simulink model "inner_pd_continuous_test"  (R2016b)
settings: Solver=VariableStepAuto  StartTime=0.0  StopTime=30  RelTol=1e-3  EnableMultiTasking=on
values from neighbouring files (symbols this model uses):
  max_ang_ref = pi/8    (= 0.392699081699)    [init.m]
  omega_max_lim = 2500    [init.m]
  omega_min_lim = 0    [init.m]
  T_max_lim = Tp - (Tp - Tm) * sat_lim    [init.m]
  tau_max_lim = 1e-5    (= 1e-05)    [init.m]
  tau_min_lim = -1e-5    (= -1e-05)    [init.m]
undefined symbols (not defined in the file or in its folder): inner_h, k
libraries: simulink x3, vrlib x2
settings Model: Creator=Daniel  LastModifiedBy=abhijit
settings DataIOCC: LimitDataPoints=on
settings OptimizationCC: LifeSpan=inf
settings DebuggingCC: AllowSymbolicDim=off  SFUnexpectedBacktrackingDiag=warning  SFNoUnconditionalDefaultTransitionDiag=warning  SFExecutionAtInitializationDiag=none
settings ModelReferenceCC: PropagateSignalLabelsOutOfModel=off
settings GRTTargetCC: TargetLangStandard=C89/C90 (ANSI)
settings ConfigComp: CovMetricSettings=dw  CovHtmlReporting=on  CovSaveCumulativeToWorkspaceVar=on  CovSaveSingleToWorkspaceVar=on  CovExternalEMLEnable=off

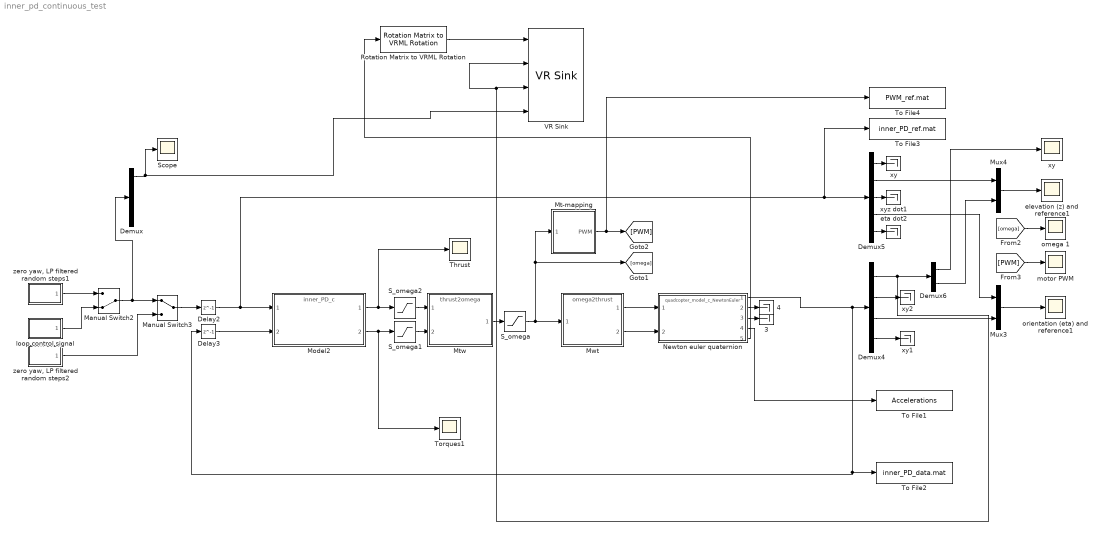
== system inner_pd_continuous_test ==
  "   3" : Terminator
  "   4" : Terminator
  "   eta dot2" : Terminator
  "   xy" : Terminator
  "   xy1" : Terminator
  "   xy2" : Terminator
  "  xyz dot1" : Terminator
  Delay2 : Delay  DelayLength=1  InitialCondition=0  SampleTime=inner_h
  Delay3 : Delay  DelayLength=1  InitialCondition=0  SampleTime=inner_h
  Demux : Demux
  Demux4 : Demux  Outputs=[3,3,3,3]
  Demux5 : Demux  Outputs=[2,1,3,3,3]
  Demux6 : Demux  Outputs=[2,1]
  Manual Switch2 : ManualSwitch  CurrentSetting=0
  Manual Switch3 : ManualSwitch
  Model2 : ModelReference  ModelNameDialog=inner_PD_c.mdl  SimulationMode=Normal  ModelReferenceVersion=1.87
  Mt-mapping : Subsystem
  Mtw : ModelReference  ModelNameDialog=thrust2omega.mdl  SimulationMode=Normal  ModelReferenceVersion=1.3
  Mux3 : Mux  Inputs=2
  Mux4 : Mux  Inputs=2
  Mwt : ModelReference  ModelNameDialog=omega2thrust.mdl  SimulationMode=Normal  ModelReferenceVersion=1.3
  Newton euler quaternion : ModelReference  ModelNameDialog=quadcopter_model_c_NewtonEuler.mdl  SimulationMode=Normal  ModelReferenceVersion=1.327
  Rotation Matrix to VRML Rotation : vrlib/Utilities/Rotation Matrix to VRML Rotation  maxzero=1e-12
  S_omega : Saturate  UpperLimit=omega_max_lim  LowerLimit=omega_min_lim
  S_omega1 : Saturate  UpperLimit=tau_max_lim  LowerLimit=tau_min_lim
  S_omega2 : Saturate  UpperLimit=T_max_lim  LowerLimit=tau_min_lim
  Scope : Scope
  Thrust : Scope
  To File1 : ToFile  Filename=Accelerations  MatrixName=Accel  SaveFormat=Timeseries  SampleTime=inner_h
  To File2 : ToFile  Filename=inner_PD_data.mat  MatrixName=PD_data  SaveFormat=Timeseries  SampleTime=inner_h
  To File3 : ToFile  Filename=inner_PD_ref.mat  MatrixName=PD_ref  SaveFormat=Timeseries  SampleTime=inner_h
  To File4 : ToFile  Filename=PWM_ref.mat  MatrixName=PWM  SaveFormat=Timeseries  SampleTime=inner_h
  Torques1 : Scope
  VR Sink : vrlib/VR Sink  InstantiateOnLoad=on  SampleTime=0.05  ViewEnable=on  RemoteChange=off  RemoteView=off  FieldsWritten=copter.rotation.4.1.1.double#copter.translation.3.1.1.double#vp.translation.3.1.1.double#target.translation.3.1.1.double  WorldFileName=copter_world.wrl  WorldDescription=quadcopter_world  AutoView=on  VideoDimensions=[]  AllowVariableSize=off  FigureProperties="{'Position', 'Name', 'Viewpoint', 'CameraBound', 'CameraDirection', 'CameraPosition', 'CameraUpVector', 'ZoomFactor', 'Antialiasing', 'Headlight', 'Lighting', 'NavPanel', 'Sound', 'StatusBar', 'Stereo3D', 'Stereo3DCameraOffset', 'Stereo3DHIT', 'ToolBar', 'Textures', 'Transparency', 'Triad', 'Wireframe', 'NavZones', 'NavMode', 'NavSpeed', 'CaptureFileFormat', 'CaptureFileName', 'Record2DCompressMethod', 'Record2DCompressQuality', 'Record2D', 'Record2DFileName', 'Record2DFPS'; [7.6000000000000000e+01   1.1600000000000000e+02   5.7600000000000000e+02   3.5000000000000000e+02], 'quadcopter_world', 'viewpoint', 'on', [0.0000000000000000e+00   0.0000000000000000e+00  -1.0000000000000000e+00], [0.0000000000000000e+00   0.0000000000000000e+00   0.0000000000000000e+00], [0.0000000000000000e+00   1.0000000000000000e+00   0.0000000000000000e+00], [1.0000000000000000e+00], 'on', 'on', 'on', 'halfbar', 'on', 'on', 'off', [1.0000000149011612e-01], [0.0000000000000000e+00], 'on', 'on', 'on', 'none', 'off', 'off', 'fly', 'normal', 'tif', '%f_anim_%n.tif', 'auto', [7.5000000000000000e+01], 'off', '%f_anim_%n.avi', 'auto'}"
  elevation (z) and reference1 : Scope
  loop control signal : Subsystem
  motor PWM : Scope
  omega 1 : Scope
  orientation (eta) and reference1 : Scope
  xy : Scope
  "zero yaw, LP filtered random steps1" : Subsystem
  "zero yaw, LP filtered random steps2" : Subsystem
  wires:
  loop control signal/1(reference) -> Manual Switch2/2
  "zero yaw, LP filtered random steps1"/1(reference) -> Manual Switch2/1
  Demux5/2 -> Mux4/1
  Mux4/1 -> elevation (z) and reference1/1
  Newton euler quaternion/1 -> Delay3/1, To File2/1, Demux4/1
  Mux3/1 -> orientation (eta) and reference1/1
  Demux5/3 -> "  xyz dot1"/1
  Demux5/5 -> "   eta dot2"/1
  Demux5/1 -> "   xy"/1
  Demux4/3 -> Mux3/2
  Demux4/1 -> VR Sink/2, VR Sink/3, Demux6/1
  [omega] -> omega 1/1
  Demux5/4 -> Mux3/1
  Delay2/1 -> Model2/1, To File3/1, Demux5/1
  Demux4/4 -> "   xy1"/1
  Demux4/2 -> "   xy2"/1
  Demux6/2 -> Mux4/2
  Demux6/1 -> xy/1
  Mt-mapping/1(PWM) -> [PWM], To File4/1
  [PWM] -> motor PWM/1
  Manual Switch2/1 -> Demux/1, Manual Switch3/1
  Manual Switch3/1 -> Delay2/1
  "zero yaw, LP filtered random steps2"/1(reference) -> Manual Switch3/2
  Newton euler quaternion/3 -> "   3"/1
  Newton euler quaternion/2 -> "   4"/1
  Mtw/1 -> S_omega/1
  Mwt/1 -> Newton euler quaternion/1
  Mwt/2 -> Newton euler quaternion/2
  S_omega/1 -> [omega], Mt-mapping/1(omega), Mwt/1
  Model2/2 -> S_omega1/1, Torques1/1
  Model2/1 -> S_omega2/1, Thrust/1
  Delay3/1 -> Model2/2
  S_omega1/1 -> Mtw/2
  S_omega2/1 -> Mtw/1
  Newton euler quaternion/4 -> To File1/1
  Demux/1 -> VR Sink/4, Scope/1
  Newton euler quaternion/5 -> Rotation Matrix to VRML Rotation/1
  Rotation Matrix to VRML Rotation/1 -> VR Sink/1

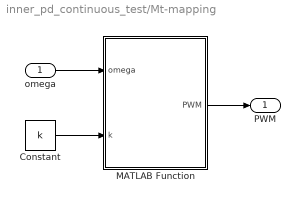
== system inner_pd_continuous_test/Mt-mapping ==
  omega : Inport
  Constant : Constant  Value=k
  MATLAB Function : MATLAB Function  TreatAsAtomicUnit=on
  PWM : Outport
  wires:
  MATLAB Function/1(PWM) -> PWM/1
  omega/1 -> MATLAB Function/1(omega)
  Constant/1 -> MATLAB Function/2(k)

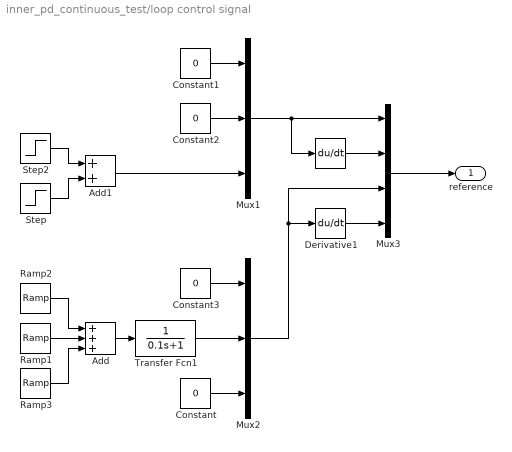
== system inner_pd_continuous_test/loop control signal ==
  "        " : Derivative
  Add : Sum  Inputs=+++
  Add1 : Sum
  Constant{,1..3} (4 alike) : Constant  Value=0
  Derivative1 : Derivative
  Mux1 : Mux  Inputs=3
  Mux2 : Mux  Inputs=3
  Mux3 : Mux  Inputs=[3,3,3,3]
  Ramp1 : simulink/Sources/Ramp  slope=2*2*pi  start=3.9  X0=0
  Ramp2 : simulink/Sources/Ramp  slope=-2*pi  start=5  X0=0
  Ramp3 : simulink/Sources/Ramp  slope=-2*pi  start=3.8  X0=0
  Step : Step  Time=5.5  After=-2  SampleTime=0
  Step2 : Step  Time=3.6  After=2  SampleTime=0
  Transfer Fcn1 : TransferFcn  Denominator=[0.1 1]
  reference : Outport
  wires:
  Mux1/1 -> "        "/1, Mux3/1
  Mux3/1 -> reference/1
  Derivative1/1 -> Mux3/4
  "        "/1 -> Mux3/2
  Mux2/1 -> Mux3/3, Derivative1/1
  Add/1 -> Transfer Fcn1/1
  Transfer Fcn1/1 -> Mux2/2
  Constant/1 -> Mux2/3
  Constant1/1 -> Mux1/1
  Constant2/1 -> Mux1/2
  Ramp2/1 -> Add/1
  Ramp1/1 -> Add/2
  Step2/1 -> Add1/1
  Step/1 -> Add1/2
  Ramp3/1 -> Add/3
  Constant3/1 -> Mux2/1
  Add1/1 -> Mux1/3

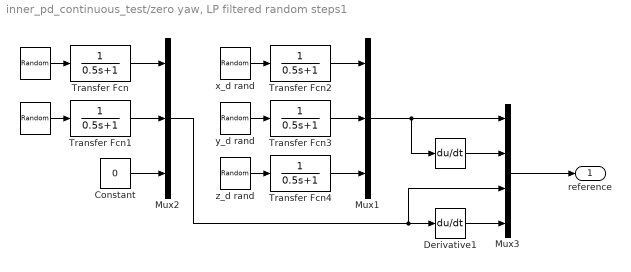
== system inner_pd_continuous_test/zero yaw, LP filtered random steps1 ==
  " " : UniformRandomNumber  Minimum=-0.2  Maximum=0.2  Seed=4  SampleTime=10
  "   " : UniformRandomNumber  Minimum=-0.2  Maximum=0.2  Seed=3  SampleTime=10
  "        " : Derivative
  Constant : Constant  Value=0
  Derivative1 : Derivative
  Mux1 : Mux  Inputs=3
  Mux2 : Mux  Inputs=3
  Mux3 : Mux  Inputs=[3,3,3,3]
  Transfer Fcn{,1..4} (5 alike) : TransferFcn  Denominator=[0.5 1]
  x_d rand : UniformRandomNumber  Minimum=-5  Maximum=5  SampleTime=10
  y_d rand : UniformRandomNumber  Minimum=-5  Maximum=5  Seed=1  SampleTime=10
  z_d rand : UniformRandomNumber  Minimum=0  Maximum=3  Seed=2  SampleTime=10
  reference : Outport
  wires:
  Mux1/1 -> "        "/1, Mux3/1
  Mux3/1 -> reference/1
  Derivative1/1 -> Mux3/4
  "        "/1 -> Mux3/2
  Mux2/1 -> Mux3/3, Derivative1/1
  "   "/1 -> Transfer Fcn/1
  " "/1 -> Transfer Fcn1/1
  Transfer Fcn/1 -> Mux2/1
  Transfer Fcn1/1 -> Mux2/2
  Constant/1 -> Mux2/3
  x_d rand/1 -> Transfer Fcn2/1
  y_d rand/1 -> Transfer Fcn3/1
  z_d rand/1 -> Transfer Fcn4/1
  Transfer Fcn2/1 -> Mux1/1
  Transfer Fcn3/1 -> Mux1/2
  Transfer Fcn4/1 -> Mux1/3

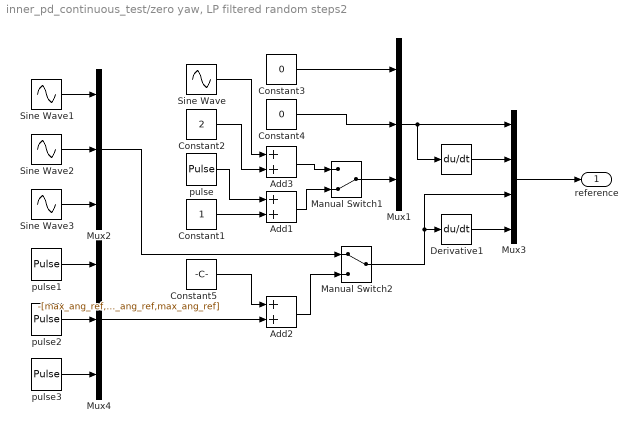
== system inner_pd_continuous_test/zero yaw, LP filtered random steps2 ==
  "        " : Derivative
  Add1 : Sum
  Add2 : Sum
  Add3 : Sum
  Constant1 : Constant
  Constant2 : Constant  Value=2
  Constant3 : Constant  Value=0
  Constant4 : Constant  Value=0
  Constant5 : Constant  Value=-[max_ang_ref,max_ang_ref,max_ang_ref]
  Derivative1 : Derivative
  Manual Switch1 : ManualSwitch  CurrentSetting=0
  Manual Switch2 : ManualSwitch
  Mux1 : Mux  Inputs=3
  Mux2 : Mux  Inputs=3
  Mux3 : Mux  Inputs=[3,3,3,3]
  Mux4 : Mux  Inputs=3
  Sine Wave : Sin  SampleTime=0
  Sine Wave1 : Sin  Amplitude=max_ang_ref  SampleTime=0
  Sine Wave2 : Sin  Amplitude=max_ang_ref  Phase=pi/2
  Sine Wave3 : Sin  Amplitude=max_ang_ref  Phase=pi  SampleTime=0
  pulse : DiscretePulseGenerator  PulseType=Time based  Amplitude=2  Period=10  PulseWidth=50
  pulse1 : DiscretePulseGenerator  PulseType=Time based  Amplitude=max_ang_ref*2  Period=10  PulseWidth=50
  pulse2 : DiscretePulseGenerator  PulseType=Time based  Amplitude=max_ang_ref*2  Period=10  PulseWidth=50
  pulse3 : DiscretePulseGenerator  PulseType=Time based  Amplitude=max_ang_ref*2  Period=10  PulseWidth=50
  reference : Outport
  wires:
  Mux1/1 -> "        "/1, Mux3/1
  Mux3/1 -> reference/1
  Derivative1/1 -> Mux3/4
  "        "/1 -> Mux3/2
  Sine Wave1/1 -> Mux2/1
  Sine Wave2/1 -> Mux2/2
  Sine Wave3/1 -> Mux2/3
  Constant3/1 -> Mux1/1
  Constant4/1 -> Mux1/2
  Sine Wave/1 -> Add3/1
  Constant2/1 -> Add3/2
  Add3/1 -> Manual Switch1/1
  Manual Switch1/1 -> Mux1/3
  Add1/1 -> Manual Switch1/2
  Constant1/1 -> Add1/2
  pulse/1 -> Add1/1
  pulse1/1 -> Mux4/1
  pulse2/1 -> Mux4/2
  pulse3/1 -> Mux4/3
  Constant5/1 -> Add2/1
  Mux4/1 -> Add2/2
  Mux2/1 -> Manual Switch2/1
  Add2/1 -> Manual Switch2/2
  Manual Switch2/1 -> Mux3/3, Derivative1/1

== matlab function inner_pd_continuous_test/Mt-mapping/MATLAB Function ==
  data: omega input; PWM output; k input
function PWM = Mt(omega, k)
%#codegen
rotor_thrusts = k.*omega.^2;
beta1 = 0.0877;
beta2 = 0.0660;
PWM =  -beta1/(2*beta2) + sqrt((beta1/(2*beta2))^2 + rotor_thrusts/beta2);
